simulink model "Problem_16_8"  (Simulink 7.5)
settings: Solver=ode45  StartTime=0.0  StopTime=10.0  RelTol=1e-3
settings Model: Creator=Holly  LastModifiedBy=Holly

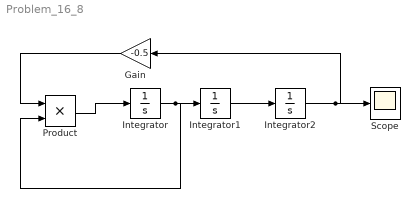
== system Problem_16_8 ==
  Gain : Gain  Gain=-0.5  ParameterDataType=fixdt(1, 16)  ParameterScaling=2^0  OutDataType=fixdt(1, 16)  OutScaling=2^0
  Integrator : Integrator  InitialCondition=0.332
  Integrator1 : Integrator
  Integrator2 : Integrator
  Product : Product  OutDataType=fixdt(1, 16)  OutScaling=2^0  RndMeth=Zero
  Scope : Scope
  wires:
  Integrator/1 -> Integrator1/1, Product/2
  Integrator1/1 -> Integrator2/1
  Integrator2/1 -> Gain/1, Scope/1
  Product/1 -> Integrator/1
  Gain/1 -> Product/1
